simulink model "mechanization_flat_earth"  (R2024a)
settings: Solver=VariableStepAuto  StartTime=0.0  StopTime=time(end)  RelTol=1e-3
values from neighbouring files (symbols this model uses):
  pos = pos_f    [test_traj_gen_v2 1.m]    (also in test_traj_gen_v2.m)
  pqr = omega_n    [test_traj_gen_v2 1.m]    (also in test_traj_gen_v2.m)
  rpy = zeros(length(time),3)    [test_traj_gen_v2 1.m]    (also in test_traj_gen_v2.m)
  ST = 1/100    (= 0.01)    [test_traj_gen_v2 1.m]    (also in test_traj_gen_v2.m)
  vel_n = vel_n_f    [test_traj_gen_v2 1.m]    (also in test_traj_gen_v2.m)
undefined symbols (not defined in the file or in its folder): DiscIntNeverNeededParam
settings Model: Creator=Lorenzo  LastModifiedBy=Lorenzo
settings RTWCC: GPUComputeCapability=3.5

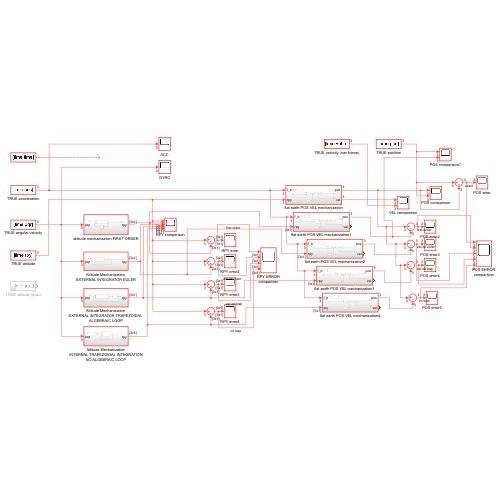
[thumbnail: Simulink's stored preview of the top-level diagram]
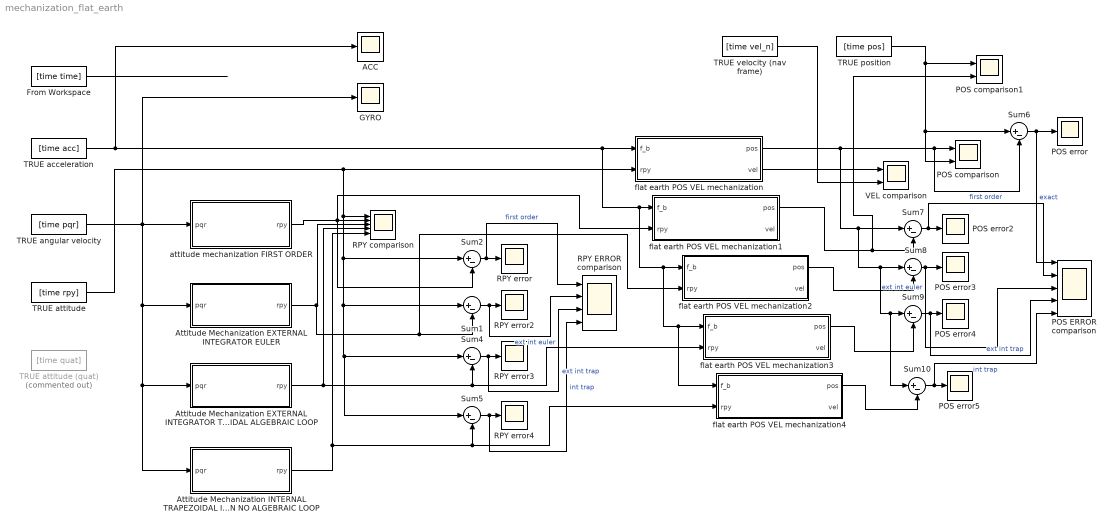
== system mechanization_flat_earth ==
  ACC : Scope
  Attitude Mechanization INTERNAL TRAPEZOIDAL INTEGRATION NO ALGEBRAIC LOOP : Subsystem
  Attitude Mechanization EXTERNAL INTEGRATOR EULER : Subsystem
  Attitude Mechanization EXTERNAL INTEGRATOR TRAPEZOIDAL ALGEBRAIC LOOP : Subsystem
  From Workspace : FromWorkspace  VariableName=[time time]  SampleTime=ST
  GYRO : Scope
  POS ERROR comparison : Scope  NumInputPorts=5
  POS comparison : Scope  NumInputPorts=2
  POS comparison1 : Scope  NumInputPorts=2
  POS error{,2..5} (5 alike) : Scope
  RPY ERROR comparison : Scope  NumInputPorts=4
  RPY comparison : Scope  NumInputPorts=5
  RPY error{,2..4} (4 alike) : Scope
  Sum{1..2,4..10} (9 alike) : Sum  Inputs=|+-
  TRUE acceleration : FromWorkspace  VariableName=[time acc]  SampleTime=ST
  TRUE angular velocity : FromWorkspace  VariableName=[time pqr]  SampleTime=ST
  TRUE attitude : FromWorkspace  VariableName=[time rpy]  SampleTime=ST
  TRUE attitude (quat) : FromWorkspace  Commented=on  VariableName=[time quat]
  TRUE position : FromWorkspace  VariableName=[time pos]  SampleTime=ST
  TRUE velocity (nav frame) : FromWorkspace  VariableName=[time vel_n]  SampleTime=ST
  VEL comparison : Scope  NumInputPorts=2
  attitude mechanization FIRST ORDER : Subsystem
  flat earth POS VEL mechanization : Subsystem
  flat earth POS VEL mechanization1 : Subsystem
  flat earth POS VEL mechanization2 : Subsystem
  flat earth POS VEL mechanization3 : Subsystem
  flat earth POS VEL mechanization4 : Subsystem
  wires:
  From Workspace/1 -> ?
  TRUE position/1 -> POS comparison1/1, Sum6/1, POS comparison/2
  TRUE velocity (nav frame)/1 -> VEL comparison/2
  Sum2/1 -> RPY ERROR comparison/1, RPY error/1  "first order"
  TRUE acceleration/1 -> ACC/1, flat earth POS VEL mechanization4/1(f_b), flat earth POS VEL mechanization3/1(f_b), flat earth POS VEL mechanization2/1(f_b), flat earth POS VEL mechanization1/1(f_b), flat earth POS VEL mechanization/1(f_b)
  flat earth POS VEL mechanization/1(pos) -> Sum10/1, Sum9/1, Sum8/1, Sum7/1, Sum6/2, POS comparison/1
  flat earth POS VEL mechanization/2(vel) -> VEL comparison/1
  TRUE angular velocity/1 -> GYRO/1, Attitude Mechanization INTERNAL TRAPEZOIDAL INTEGRATION NO ALGEBRAIC LOOP/1(pqr), Attitude Mechanization EXTERNAL INTEGRATOR TRAPEZOIDAL ALGEBRAIC LOOP/1(pqr), Attitude Mechanization EXTERNAL INTEGRATOR EULER/1(pqr), attitude mechanization FIRST ORDER/1(pqr)
  attitude mechanization FIRST ORDER/1(rpy) -> flat earth POS VEL mechanization1/2(rpy), Sum2/2, RPY comparison/2
  Attitude Mechanization EXTERNAL INTEGRATOR EULER/1(rpy) -> flat earth POS VEL mechanization2/2(rpy), Sum1/2, RPY comparison/3
  Sum1/1 -> RPY ERROR comparison/2, RPY error2/1  "ext int euler"
  Sum4/1 -> RPY ERROR comparison/3, RPY error3/1  "ext int trap"
  Attitude Mechanization EXTERNAL INTEGRATOR TRAPEZOIDAL ALGEBRAIC LOOP/1(rpy) -> flat earth POS VEL mechanization3/2(rpy), Sum4/2, RPY comparison/4
  Attitude Mechanization INTERNAL TRAPEZOIDAL INTEGRATION NO ALGEBRAIC LOOP/1(rpy) -> flat earth POS VEL mechanization4/2(rpy), Sum5/2, RPY comparison/5
  Sum5/1 -> RPY ERROR comparison/4, RPY error4/1  "int trap"
  TRUE attitude/1 -> Sum5/1, Sum4/1, Sum1/1, Sum2/1, RPY comparison/1, flat earth POS VEL mechanization/2(rpy)
  Sum6/1 -> POS ERROR comparison/1, POS error/1  "exact"
  Sum7/1 -> POS ERROR comparison/2, POS error2/1  "first order"
  flat earth POS VEL mechanization1/1(pos) -> POS comparison1/2, Sum7/2
  Sum8/1 -> POS ERROR comparison/3, POS error3/1  "ext int euler"
  flat earth POS VEL mechanization2/1(pos) -> Sum8/2
  Sum9/1 -> POS ERROR comparison/4, POS error4/1  "ext int trap"
  flat earth POS VEL mechanization3/1(pos) -> Sum9/2
  Sum10/1 -> POS ERROR comparison/5, POS error5/1  "int trap"
  flat earth POS VEL mechanization4/1(pos) -> Sum10/2

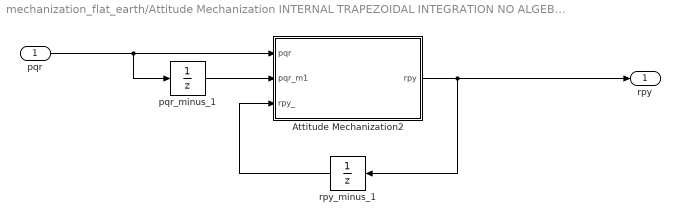
== system mechanization_flat_earth/Attitude Mechanization INTERNAL TRAPEZOIDAL INTEGRATION NO ALGEBRAIC LOOP ==
  pqr : Inport
  Attitude Mechanization2 : MATLAB Function  TreatAsAtomicUnit=on
  pqr_minus_1 : UnitDelay  InitialCondition=pqr(1,:)'  SampleTime=-1  HasFrameUpgradeWarning=on
  rpy_minus_1 : UnitDelay  InitialCondition=rpy(1,:)'  SampleTime=-1  HasFrameUpgradeWarning=on
  rpy : Outport
  wires:
  Attitude Mechanization2/1(rpy) -> rpy_minus_1/1, rpy/1
  rpy_minus_1/1 -> Attitude Mechanization2/3(rpy_)
  pqr/1 -> pqr_minus_1/1, Attitude Mechanization2/1(pqr)
  pqr_minus_1/1 -> Attitude Mechanization2/2(pqr_m1)

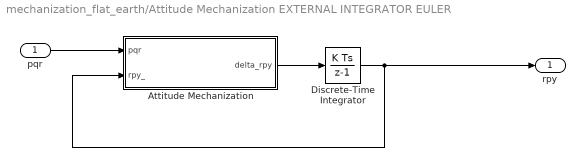
== system mechanization_flat_earth/Attitude Mechanization EXTERNAL INTEGRATOR EULER ==
  pqr : Inport
  Attitude Mechanization : MATLAB Function  TreatAsAtomicUnit=on
  Discrete-Time Integrator : DiscreteIntegrator  InitialCondition=rpy(1,:)'  SampleTime=ST  ICPrevOutput=DiscIntNeverNeededParam  ICPrevScaledInput=DiscIntNeverNeededParam
  rpy : Outport
  wires:
  Discrete-Time Integrator/1 -> rpy/1, Attitude Mechanization/2(rpy_)
  pqr/1 -> Attitude Mechanization/1(pqr)
  Attitude Mechanization/1(delta_rpy) -> Discrete-Time Integrator/1

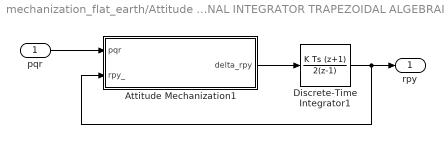
== system mechanization_flat_earth/Attitude Mechanization EXTERNAL INTEGRATOR TRAPEZOIDAL ALGEBRAIC LOOP ==
  pqr : Inport
  Attitude Mechanization1 : MATLAB Function  TreatAsAtomicUnit=on
  Discrete-Time Integrator1 : DiscreteIntegrator  IntegratorMethod=Integration: Trapezoidal  InitialCondition=rpy(1,:)'  SampleTime=ST  ICPrevOutput=DiscIntNeverNeededParam  ICPrevScaledInput=DiscIntNeverNeededParam
  rpy : Outport
  wires:
  Attitude Mechanization1/1(delta_rpy) -> Discrete-Time Integrator1/1
  pqr/1 -> Attitude Mechanization1/1(pqr)
  Discrete-Time Integrator1/1 -> Attitude Mechanization1/2(rpy_), rpy/1

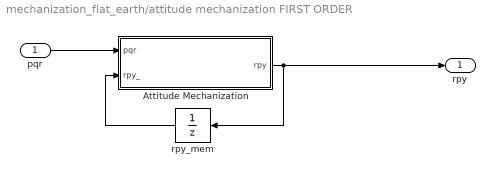
== system mechanization_flat_earth/attitude mechanization FIRST ORDER ==
  pqr : Inport
  Attitude Mechanization : MATLAB Function  TreatAsAtomicUnit=on
  rpy_mem : UnitDelay  InitialCondition=rpy(1,:)'  SampleTime=-1  HasFrameUpgradeWarning=on
  rpy : Outport
  wires:
  pqr/1 -> Attitude Mechanization/1(pqr)
  rpy_mem/1 -> Attitude Mechanization/2(rpy_)
  Attitude Mechanization/1(rpy) -> rpy_mem/1, rpy/1

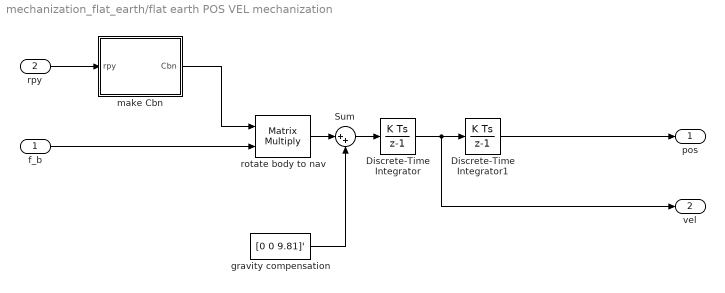
== system mechanization_flat_earth/flat earth POS VEL mechanization ==
  f_b : Inport
  rpy : Inport  Port=2
  Discrete-Time Integrator : DiscreteIntegrator  InitialCondition=vel_n(1,:)  SampleTime=-1  ICPrevOutput=DiscIntNeverNeededParam  ICPrevScaledInput=DiscIntNeverNeededParam
  Discrete-Time Integrator1 : DiscreteIntegrator  InitialCondition=pos(1,:)  SampleTime=-1  ICPrevOutput=DiscIntNeverNeededParam  ICPrevScaledInput=DiscIntNeverNeededParam
  Sum : Sum  Inputs=|++
  gravity compensation : Constant  Value=[0 0 9.81]'
  make Cbn : MATLAB Function  TreatAsAtomicUnit=on
  rotate body to nav : Product  Multiplication=Matrix(*)
  pos : Outport
  vel : Outport  Port=2
  wires:
  rotate body to nav/1 -> Sum/1
  gravity compensation/1 -> Sum/2
  Discrete-Time Integrator/1 -> vel/1, Discrete-Time Integrator1/1
  make Cbn/1(Cbn) -> rotate body to nav/1
  Discrete-Time Integrator1/1 -> pos/1
  Sum/1 -> Discrete-Time Integrator/1
  f_b/1 -> rotate body to nav/2
  rpy/1 -> make Cbn/1(rpy)

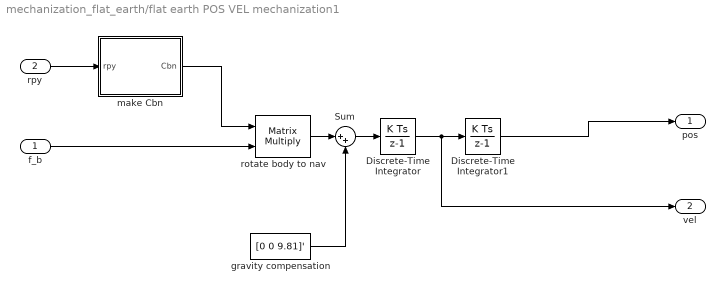
== system mechanization_flat_earth/flat earth POS VEL mechanization1 ==
  f_b : Inport
  rpy : Inport  Port=2
  Discrete-Time Integrator : DiscreteIntegrator  InitialCondition=vel_n(1,:)  SampleTime=-1  ICPrevOutput=DiscIntNeverNeededParam  ICPrevScaledInput=DiscIntNeverNeededParam
  Discrete-Time Integrator1 : DiscreteIntegrator  InitialCondition=pos(1,:)  SampleTime=-1  ICPrevOutput=DiscIntNeverNeededParam  ICPrevScaledInput=DiscIntNeverNeededParam
  Sum : Sum  Inputs=|++
  gravity compensation : Constant  Value=[0 0 9.81]'
  make Cbn : MATLAB Function  TreatAsAtomicUnit=on
  rotate body to nav : Product  Multiplication=Matrix(*)
  pos : Outport
  vel : Outport  Port=2
  wires:
  rpy/1 -> make Cbn/1(rpy)
  f_b/1 -> rotate body to nav/2
  Sum/1 -> Discrete-Time Integrator/1
  Discrete-Time Integrator1/1 -> pos/1
  make Cbn/1(Cbn) -> rotate body to nav/1
  Discrete-Time Integrator/1 -> Discrete-Time Integrator1/1, vel/1
  gravity compensation/1 -> Sum/2
  rotate body to nav/1 -> Sum/1

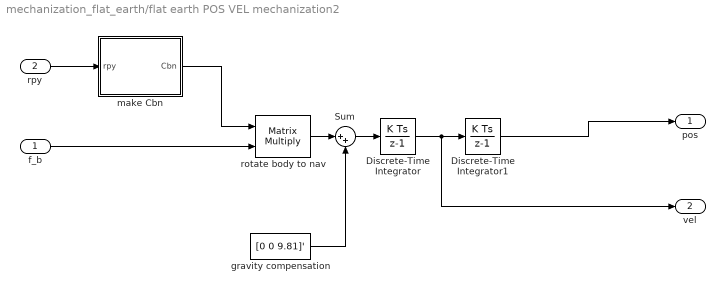
== system mechanization_flat_earth/flat earth POS VEL mechanization2 ==
  f_b : Inport
  rpy : Inport  Port=2
  Discrete-Time Integrator : DiscreteIntegrator  InitialCondition=vel_n(1,:)  SampleTime=-1  ICPrevOutput=DiscIntNeverNeededParam  ICPrevScaledInput=DiscIntNeverNeededParam
  Discrete-Time Integrator1 : DiscreteIntegrator  InitialCondition=pos(1,:)  SampleTime=-1  ICPrevOutput=DiscIntNeverNeededParam  ICPrevScaledInput=DiscIntNeverNeededParam
  Sum : Sum  Inputs=|++
  gravity compensation : Constant  Value=[0 0 9.81]'
  make Cbn : MATLAB Function  TreatAsAtomicUnit=on
  rotate body to nav : Product  Multiplication=Matrix(*)
  pos : Outport
  vel : Outport  Port=2
  wires:
  rotate body to nav/1 -> Sum/1
  gravity compensation/1 -> Sum/2
  Discrete-Time Integrator/1 -> vel/1, Discrete-Time Integrator1/1
  make Cbn/1(Cbn) -> rotate body to nav/1
  Discrete-Time Integrator1/1 -> pos/1
  Sum/1 -> Discrete-Time Integrator/1
  f_b/1 -> rotate body to nav/2
  rpy/1 -> make Cbn/1(rpy)

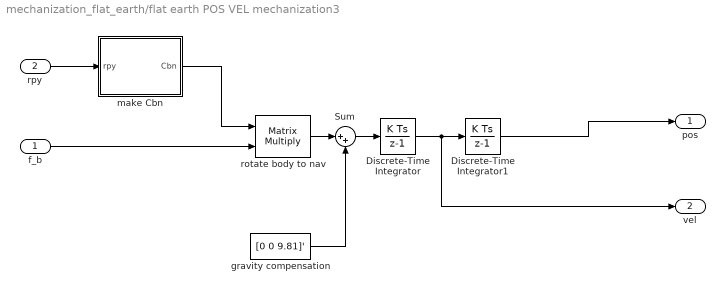
== system mechanization_flat_earth/flat earth POS VEL mechanization3 ==
  f_b : Inport
  rpy : Inport  Port=2
  Discrete-Time Integrator : DiscreteIntegrator  InitialCondition=vel_n(1,:)  SampleTime=-1  ICPrevOutput=DiscIntNeverNeededParam  ICPrevScaledInput=DiscIntNeverNeededParam
  Discrete-Time Integrator1 : DiscreteIntegrator  InitialCondition=pos(1,:)  SampleTime=-1  ICPrevOutput=DiscIntNeverNeededParam  ICPrevScaledInput=DiscIntNeverNeededParam
  Sum : Sum  Inputs=|++
  gravity compensation : Constant  Value=[0 0 9.81]'
  make Cbn : MATLAB Function  TreatAsAtomicUnit=on
  rotate body to nav : Product  Multiplication=Matrix(*)
  pos : Outport
  vel : Outport  Port=2
  wires:
  rpy/1 -> make Cbn/1(rpy)
  f_b/1 -> rotate body to nav/2
  Sum/1 -> Discrete-Time Integrator/1
  Discrete-Time Integrator1/1 -> pos/1
  make Cbn/1(Cbn) -> rotate body to nav/1
  Discrete-Time Integrator/1 -> Discrete-Time Integrator1/1, vel/1
  gravity compensation/1 -> Sum/2
  rotate body to nav/1 -> Sum/1

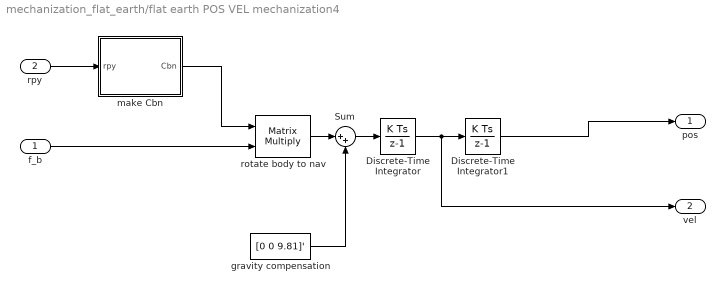
== system mechanization_flat_earth/flat earth POS VEL mechanization4 ==
  f_b : Inport
  rpy : Inport  Port=2
  Discrete-Time Integrator : DiscreteIntegrator  InitialCondition=vel_n(1,:)  SampleTime=-1  ICPrevOutput=DiscIntNeverNeededParam  ICPrevScaledInput=DiscIntNeverNeededParam
  Discrete-Time Integrator1 : DiscreteIntegrator  InitialCondition=pos(1,:)  SampleTime=-1  ICPrevOutput=DiscIntNeverNeededParam  ICPrevScaledInput=DiscIntNeverNeededParam
  Sum : Sum  Inputs=|++
  gravity compensation : Constant  Value=[0 0 9.81]'
  make Cbn : MATLAB Function  TreatAsAtomicUnit=on
  rotate body to nav : Product  Multiplication=Matrix(*)
  pos : Outport
  vel : Outport  Port=2
  wires:
  rotate body to nav/1 -> Sum/1
  gravity compensation/1 -> Sum/2
  Discrete-Time Integrator/1 -> vel/1, Discrete-Time Integrator1/1
  make Cbn/1(Cbn) -> rotate body to nav/1
  Discrete-Time Integrator1/1 -> pos/1
  Sum/1 -> Discrete-Time Integrator/1
  f_b/1 -> rotate body to nav/2
  rpy/1 -> make Cbn/1(rpy)

== matlab function mechanization_flat_earth/flat earth POS VEL mechanization1/make Cbn ==
  data: rpy input; Cbn output
function Cbn = make_Cbn(rpy)
%input:angular velocity at current timestep, latest estimation of attitude
%output> rpy and Cbn


%compute Cbn
Cz=[cos(rpy(3))     sin(rpy(3))     0; ...
    -sin(rpy(3))    cos(rpy(3))     0; ...
    0               0               1];

Cy=[cos(rpy(2))     0               -sin(rpy(2)); ...
    0               1               0; ...
    sin(rpy(2))     0               cos(rpy(2))];

Cx=[1               0               0;...
    0               cos(rpy(1))     sin(rpy(1)); ...
    0               -sin(rpy(1))    cos(rpy(1))];

Cbn = (Cx*Cy*Cz)';

== matlab function mechanization_flat_earth/attitude mechanization FIRST ORDER/Attitude Mechanization ==
  data: pqr input; rpy output; rpy_ input; ST parameter size=1
function rpy = attitude_mech(pqr,rpy_,ST)
%input:angular velocity at current timestep, latest estimation of attitude
%output> rpy and Cbn

phi = rpy_(1); 
theta = rpy_(2); 
%create Jacobian that transforms angular rates into rates of Euler
%angles
J = [1, sin(phi)*tan(theta), cos(phi)*tan(theta);
     0, cos(phi),            -sin(phi);
     0, sin(phi)/cos(theta), cos(phi)/cos(theta)];

%integrate
delta_rpy = J*pqr*ST;

rpy=rpy_ + delta_rpy;

== matlab function mechanization_flat_earth/flat earth POS VEL mechanization2/make Cbn ==
  data: rpy input; Cbn output
function Cbn = make_Cbn(rpy)
%input:angular velocity at current timestep, latest estimation of attitude
%output> rpy and Cbn


%compute Cbn
Cz=[cos(rpy(3))     sin(rpy(3))     0; ...
    -sin(rpy(3))    cos(rpy(3))     0; ...
    0               0               1];

Cy=[cos(rpy(2))     0               -sin(rpy(2)); ...
    0               1               0; ...
    sin(rpy(2))     0               cos(rpy(2))];

Cx=[1               0               0;...
    0               cos(rpy(1))     sin(rpy(1)); ...
    0               -sin(rpy(1))    cos(rpy(1))];

Cbn = (Cx*Cy*Cz)';

== matlab function mechanization_flat_earth/Attitude Mechanization EXTERNAL INTEGRATOR EULER/Attitude Mechanization ==
  data: pqr input; delta_rpy output; rpy_ input; ST parameter size=1
function delta_rpy = attitude_mech(pqr,rpy_,ST)
%input:angular velocity at current timestep, latest estimation of attitude
%output> rpy and Cbn

phi = rpy_(1); 
theta = rpy_(2); 
%create Jacobian that transforms angular rates into rates of Euler
%angles
J = [1, sin(phi)*tan(theta), cos(phi)*tan(theta);
     0, cos(phi),            -sin(phi);
     0, sin(phi)/cos(theta), cos(phi)/cos(theta)];

%integrate
delta_rpy = J*pqr;

== matlab function mechanization_flat_earth/Attitude Mechanization EXTERNAL INTEGRATOR TRAPEZOIDAL ALGEBRAIC LOOP/Attitude Mechanization1 ==
  data: pqr input; delta_rpy output; rpy_ input; ST parameter size=1
function delta_rpy = attitude_mech(pqr,rpy_,ST)
%input:angular velocity at current timestep, latest estimation of attitude
%output> rpy and Cbn

phi = rpy_(1); 
theta = rpy_(2); 
%create Jacobian that transforms angular rates into rates of Euler
%angles
J = [1, sin(phi)*tan(theta), cos(phi)*tan(theta);
     0, cos(phi),            -sin(phi);
     0, sin(phi)/cos(theta), cos(phi)/cos(theta)];

%integrate
delta_rpy = J*pqr;

== matlab function mechanization_flat_earth/flat earth POS VEL mechanization/make Cbn ==
  data: rpy input; Cbn output
function Cbn = make_Cbn(rpy)
%compute Cbn
Cz=[cos(rpy(3))     sin(rpy(3))     0; ...
    -sin(rpy(3))    cos(rpy(3))     0; ...
    0               0               1];

Cy=[cos(rpy(2))     0               -sin(rpy(2)); ...
    0               1               0; ...
    sin(rpy(2))     0               cos(rpy(2))];

Cx=[1               0               0;...
    0               cos(rpy(1))     sin(rpy(1)); ...
    0               -sin(rpy(1))    cos(rpy(1))];

Cbn = (Cx*Cy*Cz)';

== matlab function mechanization_flat_earth/Attitude Mechanization INTERNAL TRAPEZOIDAL INTEGRATION NO ALGEBRAIC LOOP/Attitude Mechanization2 ==
  data: pqr input; pqr_m1 input; rpy output; rpy_ input; ST parameter size=1
function rpy = attitude_mech(pqr, pqr_m1,rpy_,ST)
%input:angular velocity at current timestep, latest estimation of attitude
%output> rpy and Cbn

phi = rpy_(1); 
theta = rpy_(2); 
%create Jacobian that transforms angular rates into rates of Euler
%angles
J = [1, sin(phi)*tan(theta), cos(phi)*tan(theta);
     0, cos(phi),            -sin(phi);
     0, sin(phi)/cos(theta), cos(phi)/cos(theta)];
delta_rpy_m1 = J*pqr_m1*ST;

%integrate one step forward
rpy=rpy_ + delta_rpy_m1;

%get new euler angles and compute angle derivatives one step forward 
phi = rpy(1); 
theta = rpy(2); 
%create Jacobian that transforms angular rates into rates of Euler
%angles
J = [1, sin(phi)*tan(theta), cos(phi)*tan(theta);
     0, cos(phi),            -sin(phi);
     0, sin(phi)/cos(theta), cos(phi)/cos(theta)];
delta_rpy=J*pqr*ST;

%perform trapezoidal integration
rpy=rpy_ + (delta_rpy + delta_rpy_m1)/2;

== matlab function mechanization_flat_earth/flat earth POS VEL mechanization3/make Cbn ==
  data: rpy input; Cbn output
function Cbn = make_Cbn(rpy)
%input:angular velocity at current timestep, latest estimation of attitude
%output> rpy and Cbn


%compute Cbn
Cz=[cos(rpy(3))     sin(rpy(3))     0; ...
    -sin(rpy(3))    cos(rpy(3))     0; ...
    0               0               1];

Cy=[cos(rpy(2))     0               -sin(rpy(2)); ...
    0               1               0; ...
    sin(rpy(2))     0               cos(rpy(2))];

Cx=[1               0               0;...
    0               cos(rpy(1))     sin(rpy(1)); ...
    0               -sin(rpy(1))    cos(rpy(1))];

Cbn = (Cx*Cy*Cz)';

== matlab function mechanization_flat_earth/flat earth POS VEL mechanization4/make Cbn ==
  data: rpy input; Cbn output
function Cbn = make_Cbn(rpy)
%input:angular velocity at current timestep, latest estimation of attitude
%output> rpy and Cbn


%compute Cbn
Cz=[cos(rpy(3))     sin(rpy(3))     0; ...
    -sin(rpy(3))    cos(rpy(3))     0; ...
    0               0               1];

Cy=[cos(rpy(2))     0               -sin(rpy(2)); ...
    0               1               0; ...
    sin(rpy(2))     0               cos(rpy(2))];

Cx=[1               0               0;...
    0               cos(rpy(1))     sin(rpy(1)); ...
    0               -sin(rpy(1))    cos(rpy(1))];

Cbn = (Cx*Cy*Cz)';
